simulink model "SailingYachtModel3"  (R2014a)
settings: Solver=ode3  StartTime=0.0  StopTime=40  FixedStep=0.1  RelTol=1e-3
values from neighbouring files (symbols this model uses):
  alphacoeff_xdata = alphacoeff_xdata2    [param.m]
  alphacoeff_yddata = interp1(alphacoeff_xdata,alphacoeff_yddata,alphacoeff_xdata2,'pchip')    [param.m]
  alphacoeff_yldata = interp1(alphacoeff_xdata,alphacoeff_yldata,alphacoeff_xdata2,'pchip')    [param.m]
  hull_xdata = hull_xdata2    [param.m]
  hull_ydata = arrayfun(@(x)resistancehull(x),hull_xdata2)    [param.m]
  keelcoeff_xdata = keelcoeff_xdata2    [param.m]
  keelcoeff_yddata = interp1(keelcoeff_xdata,keelcoeff_yddata,keelcoeff_xdata2,'pchip')    [param.m]
  keelcoeff_yldata = interp1(keelcoeff_xdata,keelcoeff_yldata,keelcoeff_xdata2,'pchip')    [param.m]
  ruddercoeff_xdata = ruddercoeff_xdata2    [param.m]
  ruddercoeff_yddata = arrayfun(@(x)ruddercoef_cdr(x),ruddercoeff_xdata2)    [param.m]
  ruddercoeff_yldata = interp1(ruddercoeff_xdata,ruddercoeff_yldata,ruddercoeff_xdata2,'pchip')    [param.m]
undefined symbols (not defined in the file or in its folder): par
libraries: vrlib x1
settings Model: Creator=Administrator  LastModifiedBy=paul
settings DataIOCC: SignalLoggingSaveFormat=ModelDataLogs
settings OptimizationCC: ExpressionDepthLimit=2147483647  InitFltsAndDblsToZero=on
settings DebuggingCC: SaveWithParameterizedLinksMsg=none  UnderspecifiedInitializationDetection=Classic  SignalResolutionControl=TryResolveAllWithWarning  MultiTaskDSMMsg=warning  MultiTaskCondExecSysMsg=none  FcnCallInpInsideContextMsg=UseLocalSettings  StateNameClashWarn=warning
settings RTWCC: GenCodeOnly=on  BuildConfiguration=Faster Runs  IncludeERTFirstTime=on
settings GRTTargetCC: TargetFcnLib=ansi_tfl_tmw.mat  CombineOutputUpdateFcns=off  GRTInterface=on

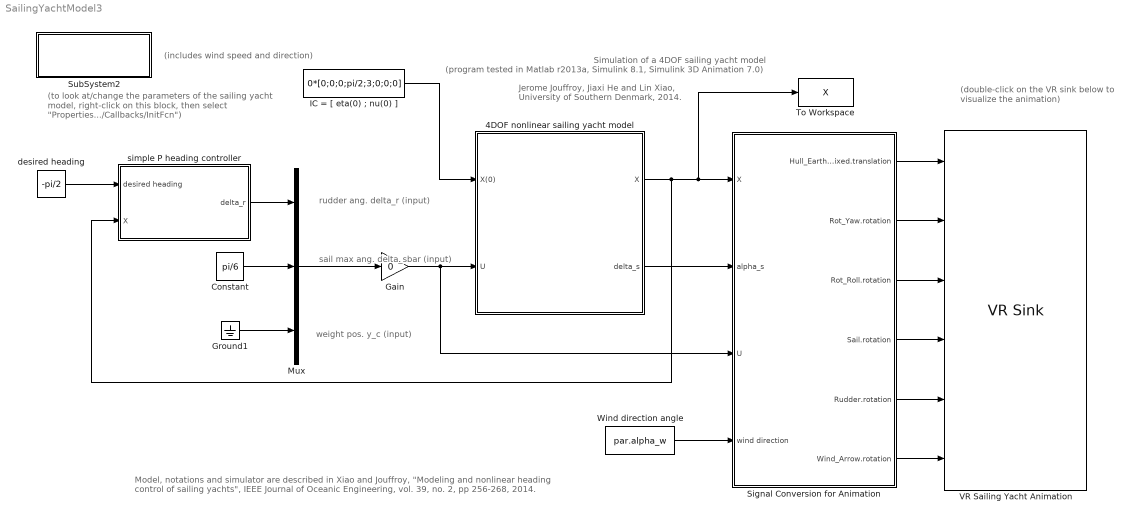
== system SailingYachtModel3 ==
  note: (includes wind speed and direction)
  note: (program tested in Matlab r2013a, Simulink 8.1, Simulink 3D Animation 7.0)
  note: (double-click on the VR sink below
      | to visualize the animation)
  note: Jerome Jouffroy, Jiaxi He and Lin Xiao,
      | University of Southern Denmark, 2014.
  note: Model, notations and simulator are described in Xiao and Jouffroy, "Modeling and nonlinear heading control of sailing yachts",
      | IEEE Journal of Oceanic Engineering, vol. 39, no. 2, pp 256-268, 2014.
  note: (to look at/change the parameters of the sailing yacht
      | model, right-click on this block, then select
      | "Properties.../Callbacks/InitFcn")
  note: weight pos. y_c (input)
  note: rudder ang. delta_r (input)
  note: sail max ang. delta_sbar (input)
  note: Simulation of a 4DOF sailing yacht model
  4DOF nonlinear sailing yacht model : Subsystem
  Constant : Constant  Value=pi/6
  Gain : Gain  Gain=0
  Ground1 : Ground
  IC = [ eta(0) ; nu(0) ] : Constant  Value=0*[0;0;0;pi/2;3;0;0;0]
  Mux : Mux  Inputs=3
  Signal Conversion for Animation : Subsystem
  SubSystem2 : Subsystem  InitFcn=|
      | global par
      | par.m = 25900;                         % (kg),mass of the vehicle
      | par.Ixx = 133690;          
      | par.Izz = 24760;      
      | par.Ixz = 2180;                        % moment of inertia
      | par.a11 = 970;   
      | par.a22 = 17430; 
      | par.a44 = 106500;
      | par.a66 = 101650;
      | par.a24 = -13160;
      | par.a26 = -6190; 
      | par.a46 = 4730;                        % (kg),added mass coef.
      | 
      | par.vt = 10;                           % the norm of wind velocity
      | par.alpha_w = pi;                      % the direction of wind (coming from the north, ie going south)
      | 
      | par.rho_a = 1.2;                       % (kg/m^3), air density
      | par.As = 170;                          % (m^2), sail area
      | par.h0 = 0.0005;                       % (m), roughness height
      | par.h1 = 11.58;                        % (m), reference height
      | par.z_s = -11.58;                      % (m), (x,y,z) is the CoE
      | par.xs = 0;
      | par.ys = 0;
      | par.zs = -11.58;                       % (m), (x,y,z) is the CoE
      | par.Xce = 0.6;                         % (m), distance along the mast to the CoE
      | par.Xm = 0.3;                          % (m), x-coordinate of the mast 
      | 
      | par.rho_w = 1025;                      % (kg/m^3), water density
      | par.Ar = 1.17;                         % (m^2), rudder area
      | par.d_r = 1.9;                         % rudder draft
      | par.zeta_r = 0.8;                      % rudder efficiency
      | par.x_r = -8.2;
      | par.z_r = -0.78;                       % (m), (x,y,z) is the CoE
      | par.xr = -8.2;
      | par.yr = 0;
      | par.zr = -0.78;                        % (m), (x,y,z) is the CoE
      | 
      | par.Ak = 8.7;                          % (m^2), keel area
      | par.d_k = 2.49;                        % keel draft
      | par.zeta_k = 0.7;                      % keel efficiency
      | par.x_k = 0;
      | par.z_k = -0.58;                       % (m), (x,y,z) is the CoE
      | par.xk = 0;
      | par.yk = 0;
      | par.zk = -0.58;                        % (m), (x,y,z) is the CoE
      | 
      | par.x_h = 0;
      | par.z_h = -1.18;                       % (m), (x,y,z) is the CoE
      | par.xh = 0;
      | par.yh = 0;
      | par.zh = -1.18;                        % (m), (x,y,z) is the CoE
      | 
      | par.w_c = 60000;                       % (N), crew weight 20000
      | par.x_c = -8;                          % (m), crew position
      | par.y_bm = 3.6;                        % (m), yacht beam
      | 
      | par.a = -5.89;
      | par.b = 8160;
      | par.c = 120000;
      | par.d = 50000;
      mask Display: disp('Parameter Initialization')
  To Workspace : ToWorkspace  VariableName=X  SaveFormat=Structure With Time  SampleTime=-1
  VR Sailing Yacht Animation : vrlib/VR Sink  InstantiateOnLoad=on  SampleTime=-1  ViewEnable=on  RemoteChange=off  RemoteView=off  FieldsWritten=Hull_EarthFixed.translation.3.1.1.double#Rot_Yaw.rotation.4.1.1.double#Rot_Roll.rotation.4.1.1.double#Sail.rotation.4.1.1.double#Rudder.rotation.4.1.1.double#Wind_Arrow.rotation.4.1.1.double  WorldFileName=SailingYachtAnimation.wrl  WorldDescription=Sailing Yacht VR animation  AutoView=on  VideoDimensions=[]  AllowVariableSize=off  FigureProperties="{'Position', 'Name', 'Viewpoint', 'CameraBound', 'CameraDirection', 'CameraPosition', 'CameraUpVector', 'ZoomFactor', 'Antialiasing', 'Headlight', 'Lighting', 'NavPanel', 'StatusBar', 'ToolBar', 'Textures', 'Transparency', 'Triad', 'Wireframe', 'NavZones', 'NavMode', 'NavSpeed', 'CaptureFileFormat', 'CaptureFileName', 'Record2DCompressMethod', 'Record2DCompressQuality', 'Record2D', 'Record2DFileName', 'Record2DFPS'; [2.0000000000000000e+00   8.0000000000000000e+01   7.9800000000000000e+02   7.1400000000000000e+02], 'Sailing Yacht VR animation', 'West', 'on', [0.0000000000000000e+00   0.0000000000000000e+00  -1.0000000000000000e+00], [0.0000000000000000e+00   0.0000000000000000e+00   0.0000000000000000e+00], [0.0000000000000000e+00   1.0000000000000000e+00   0.0000000000000000e+00], [1.0000000000000000e+00], 'on', 'on', 'on', 'halfbar', 'on', 'on', 'on', 'on', 'none', 'off', 'off', 'fly', 'normal', 'tif', '%f_anim_%n.tif', 'auto', [7.5000000000000000e+01], 'off', '%f_anim_%n.avi', 'auto'}"
  Wind direction angle : Constant  Value=par.alpha_w
  desired heading : Constant  Value=-pi/2
  simple P heading controller : Subsystem
  wires:
  Constant/1 -> Mux/2
  IC = [ eta(0) ; nu(0) ]/1 -> 4DOF nonlinear sailing yacht model/1(X(0))
  Mux/1 -> Gain/1
  4DOF nonlinear sailing yacht model/1(X) -> Signal Conversion for Animation/1(X), To Workspace/1, simple P heading controller/2(X)
  simple P heading controller/1(delta_r) -> Mux/1
  Ground1/1 -> Mux/3
  desired heading/1 -> simple P heading controller/1(desired heading)
  4DOF nonlinear sailing yacht model/2(delta_s) -> Signal Conversion for Animation/2(alpha_s)
  Wind direction angle/1 -> Signal Conversion for Animation/4(wind direction)
  Signal Conversion for Animation/1(Hull_EarthFixed.translation) -> VR Sailing Yacht Animation/1
  Signal Conversion for Animation/2(Rot_Yaw.rotation) -> VR Sailing Yacht Animation/2
  Signal Conversion for Animation/4(Sail.rotation) -> VR Sailing Yacht Animation/4
  Signal Conversion for Animation/3(Rot_Roll.rotation) -> VR Sailing Yacht Animation/3
  Signal Conversion for Animation/5(Rudder.rotation) -> VR Sailing Yacht Animation/5
  Signal Conversion for Animation/6(Wind_Arrow.rotation) -> VR Sailing Yacht Animation/6
  Gain/1 -> Signal Conversion for Animation/3(U), 4DOF nonlinear sailing yacht model/2(U)

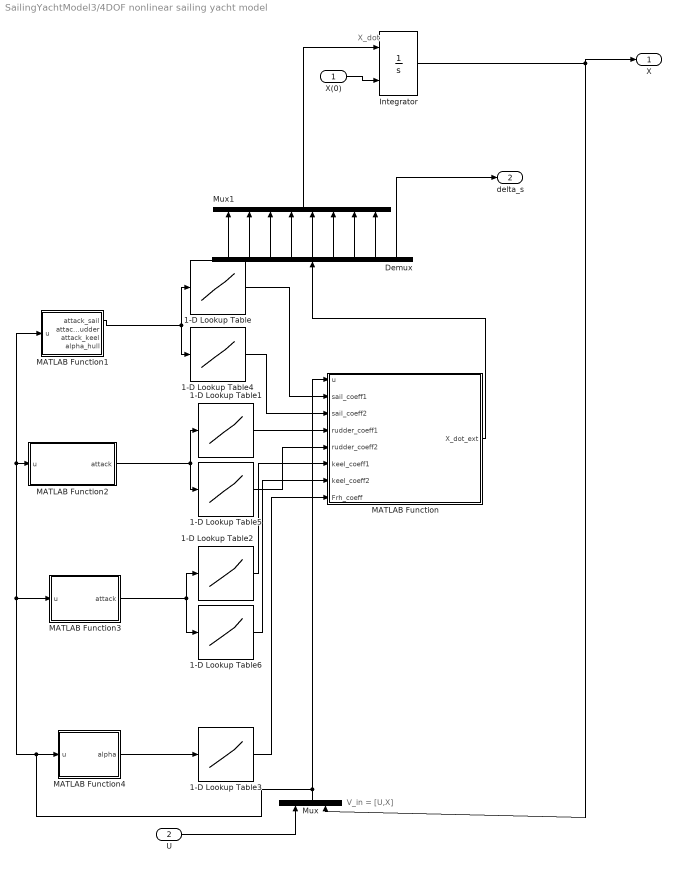
== system SailingYachtModel3/4DOF nonlinear sailing yacht model ==
  note: X_dot
  note: V_in = [U,X]
  X(0) : Inport
  U : Inport  Port=2
  1-D Lookup Table : Lookup_n-D  NumberOfTableDimensions=1  BreakpointsForDimension1=alphacoeff_xdata  Table=alphacoeff_yldata  InterpMethod=Cubic spline  RndMeth=Simplest  InputSameDT=on
  1-D Lookup Table1 : Lookup_n-D  NumberOfTableDimensions=1  BreakpointsForDimension1=ruddercoeff_xdata  Table=ruddercoeff_yldata  InterpMethod=Cubic spline  RndMeth=Simplest  InputSameDT=on
  1-D Lookup Table2 : Lookup_n-D  NumberOfTableDimensions=1  BreakpointsForDimension1=keelcoeff_xdata  Table=keelcoeff_yldata  InterpMethod=Cubic spline  DiagnosticForOutOfRangeInput=Warning  RndMeth=Simplest  InputSameDT=on
  1-D Lookup Table3 : Lookup_n-D  NumberOfTableDimensions=1  BreakpointsForDimension1=hull_xdata  Table=hull_ydata  RndMeth=Simplest  InputSameDT=on
  1-D Lookup Table4 : Lookup_n-D  NumberOfTableDimensions=1  BreakpointsForDimension1=alphacoeff_xdata  Table=alphacoeff_yddata  InterpMethod=Cubic spline  RndMeth=Simplest  InputSameDT=on
  1-D Lookup Table5 : Lookup_n-D  NumberOfTableDimensions=1  BreakpointsForDimension1=ruddercoeff_xdata  Table=ruddercoeff_yddata  InterpMethod=Cubic spline  RndMeth=Simplest  InputSameDT=on
  1-D Lookup Table6 : Lookup_n-D  NumberOfTableDimensions=1  BreakpointsForDimension1=keelcoeff_xdata  Table=keelcoeff_yddata  InterpMethod=Cubic spline  RndMeth=Simplest  InputSameDT=on
  Demux : Demux  Outputs=9
  Integrator : Integrator  InitialConditionSource=external  InitialCondition=[0;0;0;pi;1;0;0;0]
  MATLAB Function : MATLAB Function  TreatAsAtomicUnit=on
  MATLAB Function1 : MATLAB Function  TreatAsAtomicUnit=on
  MATLAB Function2 : MATLAB Function  TreatAsAtomicUnit=on
  MATLAB Function3 : MATLAB Function  TreatAsAtomicUnit=on
  MATLAB Function4 : MATLAB Function  TreatAsAtomicUnit=on
  Mux : Mux  Inputs=2
  Mux1 : Mux  Inputs=8
  X : Outport
  delta_s : Outport  Port=2
  wires:
  X(0)/1 -> Integrator/2
  Mux/1 -> MATLAB Function/1(u), MATLAB Function3/1(u), MATLAB Function2/1(u), MATLAB Function1/1(u), MATLAB Function4/1(u)
  U/1 -> Mux/1
  Integrator/1 -> X/1, Mux/2
  MATLAB Function/1(X_dot_ext) -> Demux/1
  Demux/9 -> delta_s/1
  Demux/8 -> Mux1/8
  Demux/7 -> Mux1/7
  Demux/6 -> Mux1/6
  Demux/5 -> Mux1/5
  Demux/4 -> Mux1/4
  Demux/3 -> Mux1/3
  Demux/2 -> Mux1/2
  Demux/1 -> Mux1/1
  Mux1/1 -> Integrator/1
  MATLAB Function1/1(attack_sail) -> 1-D Lookup Table/1, 1-D Lookup Table4/1
  1-D Lookup Table/1 -> MATLAB Function/2(sail_coeff1)
  MATLAB Function2/1(attack) -> 1-D Lookup Table5/1, 1-D Lookup Table1/1
  1-D Lookup Table1/1 -> MATLAB Function/4(rudder_coeff1)
  MATLAB Function3/1(attack) -> 1-D Lookup Table2/1, 1-D Lookup Table6/1
  MATLAB Function4/1(alpha) -> 1-D Lookup Table3/1
  1-D Lookup Table3/1 -> MATLAB Function/8(Frh_coeff)
  1-D Lookup Table4/1 -> MATLAB Function/3(sail_coeff2)
  1-D Lookup Table5/1 -> MATLAB Function/5(rudder_coeff2)
  1-D Lookup Table6/1 -> MATLAB Function/7(keel_coeff2)
  1-D Lookup Table2/1 -> MATLAB Function/6(keel_coeff1)

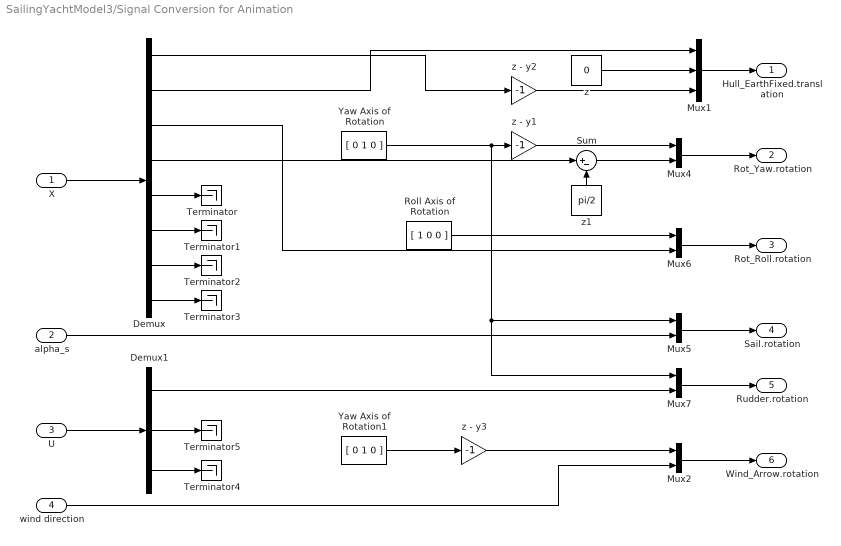
== system SailingYachtModel3/Signal Conversion for Animation ==
  X : Inport
  alpha_s : Inport  Port=2
  U : Inport  Port=3
  wind direction : Inport  Port=4
  Demux : Demux  Outputs=8
  Demux1 : Demux  Outputs=3
  Mux1 : Mux  Inputs=3
  Mux{2,4..7} (5 alike) : Mux  Inputs=2
  Roll Axis of Rotation : Constant  Value=[ 1 0 0 ]
  Sum : Sum  Inputs=|+-  SaturateOnIntegerOverflow=on
  Terminator{,1..5} (6 alike) : Terminator
  Yaw Axis of Rotation : Constant  Value=[ 0 1 0 ]
  Yaw Axis of Rotation1 : Constant  Value=[ 0 1 0 ]
  z : Constant  Value=0
  z - y1 : Gain  Gain=-1
  z - y2 : Gain  Gain=-1
  z - y3 : Gain  Gain=-1
  z1 : Constant  Value=pi/2
  Hull_EarthFixed.translation : Outport
  Rot_Yaw.rotation : Outport  Port=2
  Rot_Roll.rotation : Outport  Port=3
  Sail.rotation : Outport  Port=4
  Rudder.rotation : Outport  Port=5
  Wind_Arrow.rotation : Outport  Port=6
  wires:
  Demux/4 -> Sum/1
  Yaw Axis of Rotation/1 -> Mux5/1, Mux7/1, z - y1/1
  Sum/1 -> Mux4/2
  Roll Axis of Rotation/1 -> Mux6/1
  Demux/3 -> Mux6/2
  alpha_s/1 -> Mux5/2
  Demux/1 -> z - y2/1
  z - y2/1 -> Mux1/3
  Demux/2 -> Mux1/1
  z/1 -> Mux1/2
  z - y1/1 -> Mux4/1
  z1/1 -> Sum/2
  Mux1/1 -> Hull_EarthFixed.translation/1
  Demux/5 -> Terminator/1
  Demux/6 -> Terminator1/1
  Demux/7 -> Terminator2/1
  Demux/8 -> Terminator3/1
  X/1 -> Demux/1
  Demux1/3 -> Terminator4/1
  Demux1/2 -> Terminator5/1
  U/1 -> Demux1/1
  Demux1/1 -> Mux7/2
  Mux7/1 -> Rudder.rotation/1
  Mux5/1 -> Sail.rotation/1
  Mux4/1 -> Rot_Yaw.rotation/1
  Yaw Axis of Rotation1/1 -> z - y3/1
  z - y3/1 -> Mux2/1
  wind direction/1 -> Mux2/2
  Mux2/1 -> Wind_Arrow.rotation/1
  Mux6/1 -> Rot_Roll.rotation/1

== system SailingYachtModel3/SubSystem2 ==

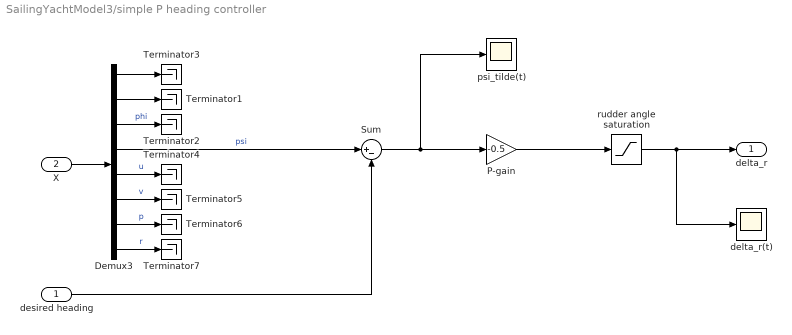
== system SailingYachtModel3/simple P heading controller ==
  desired heading : Inport
  X : Inport  Port=2
  Demux3 : Demux  Outputs=8
  P-gain : Gain  Gain=-0.5
  Sum : Sum  Inputs=|+-  SaturateOnIntegerOverflow=on
  Terminator{1..7} (7 alike) : Terminator
  delta_r(t) : Scope
      settings: YMin=-1.1  YMax=0
  psi_tilde(t) : Scope
      settings: YMin=5.55112e-17  YMax=1.6
  rudder angle saturation : Saturate  UpperLimit=pi/3  LowerLimit=-pi/3  LinearizeAsGain=off
  delta_r : Outport
  wires:
  Demux3/4 -> Sum/1  "psi"
  X/1 -> Demux3/1
  Demux3/1 -> Terminator3/1
  Demux3/2 -> Terminator1/1
  Demux3/3 -> Terminator2/1  "phi"
  Demux3/5 -> Terminator4/1  "u"
  Demux3/6 -> Terminator5/1  "v"
  Demux3/7 -> Terminator6/1  "p"
  Demux3/8 -> Terminator7/1  "r"
  Sum/1 -> psi_tilde(t)/1, P-gain/1
  P-gain/1 -> rudder angle saturation/1
  rudder angle saturation/1 -> delta_r(t)/1, delta_r/1
  desired heading/1 -> Sum/2

== matlab function SailingYachtModel3/4DOF nonlinear sailing yacht model/MATLAB Function1 ==
  data: u input; attack_sail output; attack_rudder output; attack_keel output; alpha_hull output
% interpreted Matlab function "f.m" for the Simulink file "SailingYachtModel.slx"
% This function describes the dynamics of a 4DOF sailing yacht model
% and gives the derivative of the state X and the sail angle delta_s.
% The input vector V_in contains the system state and the control input vector. 
%
% For the model description, notations, equations and parameters,
% see Xiao and Jouffroy, "Modeling and nonlinear heading control of sailing
% yachts", IEEE Journal of Oceanic Engineering, vol. 39, no. 2., pp. 256-268, 2014.
% 
% Jerome Jouffroy, Jiaxi He and Lin Xiao, 2014.
% University of Southern Denmark.



function [attack_sail,attack_rudder,attack_keel,alpha_hull]=sailcoeff_attack(u)
%#codegen

% use the system parameters
par = modeleBoat();

V_in = u;
% retrieve the system state from the field input vector "V_in"
x = V_in(5);
y = V_in(6);
phi = V_in(7);
psi = V_in(8);
u = V_in(9);
v = V_in(10);
p = V_in(11);
r = V_in(12);
nu = [ u ; v ; p ; r ];

% retrieve the input signals from the vector "V_in"
delta_r = V_in(1);
delta_sbar = V_in(2);
y_w = V_in(3);
u_s = V_in(4);


% evaluate the matrix M and C in the model
M_RB = [ par.m 0 0 0 ; 0 par.m 0 0 ; 0 0 par.Ixx -par.Ixz ; 0 0 -par.Ixz par.Izz];
C_RB = [0 -par.m*r 0 0 ; par.m*r 0 0 0 ; 0 0 0 0 ; 0 0 0 0];

M_A = [par.a11 0 0 0;0 par.a22 par.a24 par.a26;0 par.a24 par.a44 par.a46;0 par.a26 par.a46 par.a66];
C_A = [0  0 0 -par.a22*nu(2)-par.a24*nu(3)-par.a26*nu(4) ; 0 0 0 par.a11*nu(1) ; 0 0 0 0 ; par.a22*nu(2)+par.a24*nu(3)+par.a26*nu(4) -par.a11*nu(1) 0 0];

M = M_RB + M_A;

% calculate the tau vector, ie forces and moments generated from:
% the sail
v_t = [ par.vt*cos(par.alpha_w); par.vt*sin(par.alpha_w); 0 ];
v_tw = log(abs(par.z_s)*cos(phi)/par.h0)/log(par.h1/par.h0)*v_t;
R1 = [ cos(-psi) -sin(-psi) 0; sin(-psi) cos(-psi) 0; 0 0 1];
R2 = [ 1 0 0 ; 0 cos(-phi) -sin(-phi); 0 sin(-phi) cos(-phi)];
v_tb = R2*R1*v_tw; % wind expressed in the body frame
V_in = [ u ; v ; 0 ];
V_awb = v_tb - V_in - cross([p;0;r],[par.xs;par.ys;par.zs]);
V_awu = V_awb(1);
V_awv = V_awb(2);
alpha_aw = atan2(V_awv,-V_awu);

%% (sail luffing or not)
if alpha_aw-u_s>delta_sbar
    delta_s = delta_sbar;
elseif alpha_aw-u_s<-delta_sbar
    delta_s = -delta_sbar;
else
    delta_s = alpha_aw-u_s;
end
delta_s = delta_s + u_s;

alpha_as = alpha_aw - delta_s;

attack_sail = alpha_as;

% fit the input angle of attack into the interval [-pi,pi]
if attack_sail > pi
    attack_sail = mod(attack_sail+pi,2*pi) - pi;
else
    if attack_sail < -pi
        attack_sail = mod(attack_sail-pi,-2*pi) + pi;
    end
end

%% the rudder
v_aru = -u+r*par.yr;
v_arv = -v-r*par.xr + p*par.zr;
alpha_ar = atan2(v_arv,-v_aru);
alpha_a = alpha_ar-delta_r;

attack_rudder = alpha_a;

% fit the input angle of attack into the interval [-pi,pi]
if attack_rudder > pi
    attack_rudder = mod(attack_rudder+pi,2*pi) - pi;
else
    if attack_rudder < -pi
        attack_rudder = mod(attack_rudder-pi,-2*pi) + pi;
    end
end

%% the keel
v_aku = -u + r*par.yk;
v_akv = -v - r*par.xk+p*par.zk;
alpha_ak = atan2(v_akv,-v_aku);
alpha_e = alpha_ak;

attack_keel = alpha_e;

% fit the input angle of attack into the interval [-pi,pi]
if attack_keel > pi
    attack_keel = mod(attack_keel+pi,2*pi) - pi;
else
    if attack_keel < -pi
        attack_keel = mod(attack_keel-pi,-2*pi) + pi;
    end
end

%% from the hull
v_ahu = -u + r*par.yh;
v_ahv = (-v-r*par.xh + p*par.zh)/cos(phi);
v_ah = sqrt(v_aku^2+v_akv^2);
alpha_ah = atan2(v_ahv,-v_ahu);
alpha_hull = v_ah;

== matlab function SailingYachtModel3/4DOF nonlinear sailing yacht model/MATLAB Function ==
  data: u input; X_dot_ext output; sail_coeff1 input; sail_coeff2 input; rudder_coeff1 input; rudder_coeff2 input; keel_coeff1 input; keel_coeff2 input; Frh_coeff input
% interpreted Matlab function "f.m" for the Simulink file "SailingYachtModel.slx"
% This function describes the dynamics of a 4DOF sailing yacht model
% and gives the derivative of the state X and the sail angle delta_s.
% The input vector V_in contains the system state and the control input vector. 
%
% For the model description, notations, equations and parameters,
% see Xiao and Jouffroy, "Modeling and nonlinear heading control of sailing
% yachts", IEEE Journal of Oceanic Engineering, vol. 39, no. 2., pp. 256-268, 2014.
% 
% Jerome Jouffroy, Jiaxi He and Lin Xiao, 2014.
% University of Southern Denmark.



function X_dot_ext  =fcn(u,sail_coeff1,sail_coeff2,rudder_coeff1,rudder_coeff2,keel_coeff1,keel_coeff2,Frh_coeff)
%#codegen

% use the system parameters
par = modeleBoat();

V_in = u;
% retrieve the system state from the field input vector "V_in"
x = V_in(4);
y = V_in(5);
phi = V_in(6);
psi = V_in(7);
u = V_in(8);
v = V_in(9);
p = V_in(10);
r = V_in(11);
nu = [ u ; v ; p ; r ];

% retrieve the input signals from the vector "V_in"
delta_r = V_in(1);
delta_sbar = V_in(2);
y_w = V_in(3);

% evaluate the matrix M and C in the model
M_RB = [ par.m 0 0 0 ; 0 par.m 0 0 ; 0 0 par.Ixx -par.Ixz ; 0 0 -par.Ixz par.Izz];
C_RB = [0 -par.m*r 0 0 ; par.m*r 0 0 0 ; 0 0 0 0 ; 0 0 0 0];

M_A = [par.a11 0 0 0;0 par.a22 par.a24 par.a26;0 par.a24 par.a44 par.a46;0 par.a26 par.a46 par.a66];
C_A = [0  0 0 -par.a22*nu(2)-par.a24*nu(3)-par.a26*nu(4) ; 0 0 0 par.a11*nu(1) ; 0 0 0 0 ; par.a22*nu(2)+par.a24*nu(3)+par.a26*nu(4) -par.a11*nu(1) 0 0];

M = M_RB + M_A;

% calculate the tau vector, ie forces and moments generated from:
% the sail
v_t = [ par.vt*cos(par.alpha_w); par.vt*sin(par.alpha_w); 0 ];
v_tw = log(abs(par.z_s)*cos(phi)/par.h0)/log(par.h1/par.h0)*v_t;
R1 = [ cos(-psi) -sin(-psi) 0; sin(-psi) cos(-psi) 0; 0 0 1];
R2 = [ 1 0 0 ; 0 cos(-phi) -sin(-phi); 0 sin(-phi) cos(-phi)];
v_tb = R2*R1*v_tw; % wind expressed in the body frame
V_in = [ u ; v ; 0 ];
V_awb = v_tb - V_in - cross([p;0;r],[par.xs;par.ys;par.zs]);
V_awu = V_awb(1);
V_awv = V_awb(2);
alpha_aw = atan2(V_awv,-V_awu);

% (sail luffing or not)
if alpha_aw>delta_sbar
    delta_s = delta_sbar;
elseif alpha_aw<-delta_sbar
    delta_s = -delta_sbar;
else
    delta_s = alpha_aw;
end

alpha_as = alpha_aw - delta_s;

Cls = sail_coeff1;
Cds = sail_coeff2;

Ls = 0.5*par.rho_a*par.As*(V_awu^2+V_awv^2)*Cls;
Ds = 0.5*par.rho_a*par.As*(V_awu^2+V_awv^2)*Cds;

tau_sail = [Ls*sin(alpha_aw)-Ds*cos(alpha_aw); Ls*cos(alpha_aw)+Ds*sin(alpha_aw);-(Ls*cos(alpha_aw)+Ds*sin(alpha_aw))*par.zs; -(Ls*sin(alpha_aw)-Ds*cos(alpha_aw))*par.Xce*sin(delta_s)+(Ls*cos(alpha_aw)+Ds*sin(alpha_aw))*(par.Xm-par.Xce*cos(delta_s))];
Mzs = tau_sail(4);

% the rudder
v_aru = -u+r*par.yr;
v_arv = -v-r*par.xr + p*par.zr;
alpha_ar = atan2(v_arv,-v_aru);
alpha_a = alpha_ar-delta_r;

%[Clr,Cdr] = ruddercoef(alpha_a);
Clr = rudder_coeff1;
Cdr = rudder_coeff2;

Cdr = Cdr+Clr^2*par.Ar/(pi*2*par.zeta_r*par.d_r^2);

Lr = 0.5*par.rho_w*par.Ar*(v_aru^2+v_arv^2)*Clr;
Dr = 0.5*par.rho_w*par.Ar*(v_aru^2+v_arv^2)*Cdr;

tau_rudder = [Lr*sin(alpha_ar)-Dr*cos(alpha_ar); Lr*cos(alpha_ar)+Dr*sin(alpha_ar); -(Lr*cos(alpha_ar)+Dr*sin(alpha_ar))*par.zr; (Lr*cos(alpha_ar)+Dr*sin(alpha_ar))*par.xr];
Mzr = tau_rudder(4);

% the tau vector is finally given by:
tau = tau_sail + tau_rudder;

% calculate the damping forces and moments:
% from the keel
v_aku = -u + r*par.yk;
v_akv = -v - r*par.xk+p*par.zk;
alpha_ak = atan2(v_akv,-v_aku);
alpha_e = alpha_ak;

Clk = keel_coeff1;
Cdk = keel_coeff2;

Cdk = Cdk + Clk^2*par.Ak/(pi*2*par.zeta_k*par.d_k^2);

Lk = 0.5*par.rho_w*par.Ak*(v_aku^2+v_akv^2)*Clk;
Dk = 0.5*par.rho_w*par.Ak*(v_aku^2+v_akv^2)*Cdk;

D_keel = [ -Lk*sin(alpha_ak)+Dk*cos(alpha_ak); -Lk*cos(alpha_ak)-Dk*sin(alpha_ak); -(-Lk*cos(alpha_ak)-Dk*sin(alpha_ak))*par.zk; -(Lk*cos(alpha_ak)+Dk*sin(alpha_ak))*par.xk];

% from the hull
v_ahu = -u + r*par.yh;
v_ahv = (-v-r*par.xh + p*par.zh)/cos(phi);
v_ah = sqrt(v_aku^2+v_akv^2);
alpha_ah = atan2(v_ahv,-v_ahu);

Frh = Frh_coeff;

D_hull = [Frh*cos(alpha_ah);-Frh*sin(alpha_ah)*cos(phi); Frh*sin(alpha_ah)*cos(phi)*par.zh; -Frh*sin(alpha_ah)*cos(phi)*par.xh];

% from heel and yaw
% (compute first eta_dot and thereby phi_dot and psi_dot)
J = [cos(psi) -sin(psi)*cos(phi) 0 0; sin(psi) cos(psi)*cos(phi) 0 0; 0 0 1 0; 0 0 0 cos(phi)];
eta_dot = J*nu;
phi_dot = eta_dot(3);
psi_dot = eta_dot(4);

D_heelandyaw = [0;0;par.c*phi_dot*abs(phi_dot);par.d*psi_dot*abs(psi_dot)*cos(phi)]; 

% compute total damping vector D
D = D_keel + D_hull + D_heelandyaw;

% righting moment plus internal moving mass system (ie transversal weight)
phi_deg = phi*180/pi;
M_xw = -y_w*par.w_c*par.y_bm*cos(phi);
M_zw = -y_w*par.w_c*par.x_c*sin(abs(phi));
G = [ 0 ; 0 ; par.a*phi_deg^2+par.b*phi_deg + M_xw ; M_zw];

% computation of nu_dot
nu_dot = -M\(C_RB*nu+C_A*nu)-M\D-M\G+M\tau; 
 

% output the derivative of the state extended with the sail angle
X_dot_ext = [ eta_dot   ; 
              nu_dot   ;
              delta_s];

== matlab function SailingYachtModel3/4DOF nonlinear sailing yacht model/MATLAB Function2 ==
  data: u input; attack output
% interpreted Matlab function "f.m" for the Simulink file "SailingYachtModel.slx"
% This function describes the dynamics of a 4DOF sailing yacht model
% and gives the derivative of the state X and the sail angle delta_s.
% The input vector V_in contains the system state and the control input vector. 
%
% For the model description, notations, equations and parameters,
% see Xiao and Jouffroy, "Modeling and nonlinear heading control of sailing
% yachts", IEEE Journal of Oceanic Engineering, vol. 39, no. 2., pp. 256-268, 2014.
% 
% Jerome Jouffroy, Jiaxi He and Lin Xiao, 2014.
% University of Southern Denmark.



function attack=ruddercoeff_attack(u)
%#codegen

% use the system parameters
par = modeleBoat();


V_in = u;
% retrieve the system state from the field input vector "V_in"
x = V_in(4);
y = V_in(5);
phi = V_in(6);
psi = V_in(7);
u = V_in(8);
v = V_in(9);
p = V_in(10);
r = V_in(11);
nu = [ u ; v ; p ; r ];

% retrieve the input signals from the vector "V_in"
delta_r = V_in(1);
delta_sbar = V_in(2);
y_w = V_in(3);

% evaluate the matrix M and C in the model
M_RB = [ par.m 0 0 0 ; 0 par.m 0 0 ; 0 0 par.Ixx -par.Ixz ; 0 0 -par.Ixz par.Izz];
C_RB = [0 -par.m*r 0 0 ; par.m*r 0 0 0 ; 0 0 0 0 ; 0 0 0 0];

M_A = [par.a11 0 0 0;0 par.a22 par.a24 par.a26;0 par.a24 par.a44 par.a46;0 par.a26 par.a46 par.a66];
C_A = [0  0 0 -par.a22*nu(2)-par.a24*nu(3)-par.a26*nu(4) ; 0 0 0 par.a11*nu(1) ; 0 0 0 0 ; par.a22*nu(2)+par.a24*nu(3)+par.a26*nu(4) -par.a11*nu(1) 0 0];

M = M_RB + M_A;

% calculate the tau vector, ie forces and moments generated from:
% the sail
v_t = [ par.vt*cos(par.alpha_w); par.vt*sin(par.alpha_w); 0 ];
v_tw = log(abs(par.z_s)*cos(phi)/par.h0)/log(par.h1/par.h0)*v_t;
R1 = [ cos(-psi) -sin(-psi) 0; sin(-psi) cos(-psi) 0; 0 0 1];
R2 = [ 1 0 0 ; 0 cos(-phi) -sin(-phi); 0 sin(-phi) cos(-phi)];
v_tb = R2*R1*v_tw; % wind expressed in the body frame
V_in = [ u ; v ; 0 ];
V_awb = v_tb - V_in - cross([p;0;r],[par.xs;par.ys;par.zs]);
V_awu = V_awb(1);
V_awv = V_awb(2);
alpha_aw = atan2(V_awv,-V_awu);

% (sail luffing or not)
if alpha_aw>delta_sbar
    delta_s = delta_sbar;
elseif alpha_aw<-delta_sbar
    delta_s = -delta_sbar;
else
    delta_s = alpha_aw;
end

alpha_as = alpha_aw - delta_s;


% the rudder
v_aru = -u+r*par.yr;
v_arv = -v-r*par.xr + p*par.zr;
alpha_ar = atan2(v_arv,-v_aru);
alpha_a = alpha_ar-delta_r;

attack = alpha_a;

% fit the input angle of attack into the interval [-pi,pi]
if attack > pi
    attack = mod(attack+pi,2*pi) - pi;
else
    if attack < -pi
        attack = mod(attack-pi,-2*pi) + pi;
    end
end

% interpolation
%attack = attack/pi*180;




%------------------------------------------------------------------------------------------------------------------------------
function [Clr,Cdr] = ruddercoef(attack)
% generate a lookup table for the lift/drag coefficients for the sail
% and compute Cls/Cds from the lookup table using interpolation.

% lookup table
xdata = linspace(-pi,pi,73); % every 5 degrees
xdata = xdata/pi*180;

% lift curve
yl = fliplr([0 0.42 0.73 ...
    0.95 1.1 1.165 1.18 1.155 1.12 1.065 1 0.92 0.83 0.72 0.62 0.48 0.33 0.16])*(-1);
yldata = [fliplr([0 0.42 0.73 ...
    0.95 1.1 1.165 1.18 1.155 1.12 1.065 1 0.92 0.83 0.72 0.62 0.48 0.33 0.16 0 yl])*(-1) ...
    [0.42 0.73 ...
    0.95 1.1 1.165 1.18 1.155 1.12 1.065 1 0.92 0.83 0.72 0.62 0.48 0.33 0.16 0 yl]];

% drag curve
yd = fliplr([0 0.03 0.06 ...
    0.1 0.17 0.3 0.48 0.74 0.98 1.18 1.34 1.5 1.65 1.76 1.89 1.97 2.01 2.05]);
yddata = [fliplr([0 0.03 0.06 ...
    0.1 0.17 0.3 0.48 0.74 0.98 1.18 1.34 1.5 1.65 1.76 1.89 1.97 2.01 2.05 2.08 yd])...
    [0.03 0.06 ...
    0.1 0.17 0.3 0.48 0.74 0.98 1.18 1.34 1.5 1.65 1.76 1.89 1.97 2.01 2.05 2.08 yd]];

% fit the input angle of attack into the interval [-pi,pi]
if attack > pi
    attack = mod(attack+pi,2*pi) - pi;
else
    if attack < -pi
        attack = mod(attack-pi,-2*pi) + pi;
    end
end

% interpolation
attack = attack/pi*180;
Clr = interp1(xdata,yldata,attack,'pchip');
Cdr = interp1(xdata,yddata,attack,'pchip');


%------------------------------------------------------------------------------------------------------------------------------
function [Clk,Cdk] = keelcoef(attack)
% generate a lookup table for the lift/drag coefficients for the sail
% and compute Cls/Cds from the lookup table using interpolation.

% lookup table
xdata = linspace(-pi,pi,73); % every 5 degrees
xdata = xdata/pi*180;

% lift curve
yl = fliplr([0 0.425 0.74 ...
    0.94 1.1 1.17 1.19 1.16 1.12 1.07 0.99 0.92 0.84 0.74 0.63 0.49 0.345 0.185])*(-1);
yldata = [fliplr([0 0.425 0.74 ...
    0.94 1.1 1.17 1.19 1.16 1.12 1.07 0.99 0.92 0.84 0.74 0.63 0.49 0.345 0.185 0 yl])*(-1) ...
    [0.425 0.74 ...
    0.94 1.1 1.17 1.19 1.16 1.12 1.07 0.99 0.92 0.84 0.74 0.63 0.49 0.345 0.185 0 yl]];

% drag curve
yd = fliplr([0 0.04 0.07 ...
    0.1 0.17 0.3 0.49 0.76 0.98 1.19 1.34 1.5 1.65 1.77 1.88 1.96 2.01 2.05]);
yddata = [fliplr([0 0.04 0.07 ...
    0.1 0.17 0.3 0.49 0.76 0.98 1.19 1.34 1.5 1.65 1.77 1.88 1.96 2.01 2.05 2.09 yd])...
    [0.04 0.07 ...
    0.1 0.17 0.3 0.49 0.76 0.98 1.19 1.34 1.5 1.65 1.77 1.88 1.96 2.01 2.05 2.09 yd]];

% fit the input angle of attack into the interval [-pi,pi]
if attack > pi
    attack = mod(attack+pi,2*pi) - pi;
else
    if attack < -pi
        attack = mod(attack-pi,-2*pi) + pi;
    end
end

% interpolation
attack = attack/pi*180;
Clk = interp1(xdata,yldata,attack,'pchip');
Cdk = interp1(xdata,yddata,attack,'pchip');


%------------------------------------------------------------------------------------------------------------------------------
function F = resistancehull(alpha_a)

xdata = linspace(0,6,13); % every 0.5m/s
ydata = [0 0.15 0.35 0.5 0.675 0.825 1.175 1.4 2 4.85 9.85 18.46 27.5]*1000;

% interpolation
if alpha_a <= 6
    F = interp1(xdata,ydata,alpha_a,'pchip');
else
    F = interp1(xdata,ydata,alpha_a,'pchip','extrap');
end

== matlab function SailingYachtModel3/4DOF nonlinear sailing yacht model/MATLAB Function3 ==
  data: u input; attack output
% interpreted Matlab function "f.m" for the Simulink file "SailingYachtModel.slx"
% This function describes the dynamics of a 4DOF sailing yacht model
% and gives the derivative of the state X and the sail angle delta_s.
% The input vector V_in contains the system state and the control input vector. 
%
% For the model description, notations, equations and parameters,
% see Xiao and Jouffroy, "Modeling and nonlinear heading control of sailing
% yachts", IEEE Journal of Oceanic Engineering, vol. 39, no. 2., pp. 256-268, 2014.
% 
% Jerome Jouffroy, Jiaxi He and Lin Xiao, 2014.
% University of Southern Denmark.



function attack=keelcoeff_attack(u)
%#codegen

% use the system parameters
par = modeleBoat();


V_in = u;
% retrieve the system state from the field input vector "V_in"
x = V_in(4);
y = V_in(5);
phi = V_in(6);
psi = V_in(7);
u = V_in(8);
v = V_in(9);
p = V_in(10);
r = V_in(11);
nu = [ u ; v ; p ; r ];

% retrieve the input signals from the vector "V_in"
delta_r = V_in(1);
delta_sbar = V_in(2);
y_w = V_in(3);

% evaluate the matrix M and C in the model
M_RB = [ par.m 0 0 0 ; 0 par.m 0 0 ; 0 0 par.Ixx -par.Ixz ; 0 0 -par.Ixz par.Izz];
C_RB = [0 -par.m*r 0 0 ; par.m*r 0 0 0 ; 0 0 0 0 ; 0 0 0 0];

M_A = [par.a11 0 0 0;0 par.a22 par.a24 par.a26;0 par.a24 par.a44 par.a46;0 par.a26 par.a46 par.a66];
C_A = [0  0 0 -par.a22*nu(2)-par.a24*nu(3)-par.a26*nu(4) ; 0 0 0 par.a11*nu(1) ; 0 0 0 0 ; par.a22*nu(2)+par.a24*nu(3)+par.a26*nu(4) -par.a11*nu(1) 0 0];

M = M_RB + M_A;

% calculate the tau vector, ie forces and moments generated from:
% the sail
v_t = [ par.vt*cos(par.alpha_w); par.vt*sin(par.alpha_w); 0 ];
v_tw = log(abs(par.z_s)*cos(phi)/par.h0)/log(par.h1/par.h0)*v_t;
R1 = [ cos(-psi) -sin(-psi) 0; sin(-psi) cos(-psi) 0; 0 0 1];
R2 = [ 1 0 0 ; 0 cos(-phi) -sin(-phi); 0 sin(-phi) cos(-phi)];
v_tb = R2*R1*v_tw; % wind expressed in the body frame
V_in = [ u ; v ; 0 ];
V_awb = v_tb - V_in - cross([p;0;r],[par.xs;par.ys;par.zs]);
V_awu = V_awb(1);
V_awv = V_awb(2);
alpha_aw = atan2(V_awv,-V_awu);


% calculate the damping forces and moments:
% from the keel
v_aku = -u + r*par.yk;
v_akv = -v - r*par.xk+p*par.zk;
alpha_ak = atan2(v_akv,-v_aku);
alpha_e = alpha_ak;

attack = alpha_e;

% fit the input angle of attack into the interval [-pi,pi]
if attack > pi
    attack = mod(attack+pi,2*pi) - pi;
else
    if attack < -pi
        attack = mod(attack-pi,-2*pi) + pi;
    end
end

% interpolation
%attack = attack/pi*180;

== matlab function SailingYachtModel3/4DOF nonlinear sailing yacht model/MATLAB Function4 ==
  data: u input; alpha output
% interpreted Matlab function "f.m" for the Simulink file "SailingYachtModel.slx"
% This function describes the dynamics of a 4DOF sailing yacht model
% and gives the derivative of the state X and the sail angle delta_s.
% The input vector V_in contains the system state and the control input vector. 
%
% For the model description, notations, equations and parameters,
% see Xiao and Jouffroy, "Modeling and nonlinear heading control of sailing
% yachts", IEEE Journal of Oceanic Engineering, vol. 39, no. 2., pp. 256-268, 2014.
% 
% Jerome Jouffroy, Jiaxi He and Lin Xiao, 2014.
% University of Southern Denmark.



function alpha=fcn(u)
%#codegen

% use the system parameters
par = modeleBoat();


V_in = u;
% retrieve the system state from the field input vector "V_in"
x = V_in(4);
y = V_in(5);
phi = V_in(6);
psi = V_in(7);
u = V_in(8);
v = V_in(9);
p = V_in(10);
r = V_in(11);
nu = [ u ; v ; p ; r ];

% retrieve the input signals from the vector "V_in"
delta_r = V_in(1);
delta_sbar = V_in(2);
y_w = V_in(3);

% evaluate the matrix M and C in the model
M_RB = [ par.m 0 0 0 ; 0 par.m 0 0 ; 0 0 par.Ixx -par.Ixz ; 0 0 -par.Ixz par.Izz];
C_RB = [0 -par.m*r 0 0 ; par.m*r 0 0 0 ; 0 0 0 0 ; 0 0 0 0];

M_A = [par.a11 0 0 0;0 par.a22 par.a24 par.a26;0 par.a24 par.a44 par.a46;0 par.a26 par.a46 par.a66];
C_A = [0  0 0 -par.a22*nu(2)-par.a24*nu(3)-par.a26*nu(4) ; 0 0 0 par.a11*nu(1) ; 0 0 0 0 ; par.a22*nu(2)+par.a24*nu(3)+par.a26*nu(4) -par.a11*nu(1) 0 0];

M = M_RB + M_A;

% calculate the tau vector, ie forces and moments generated from:
% the sail
v_t = [ par.vt*cos(par.alpha_w); par.vt*sin(par.alpha_w); 0 ];
v_tw = log(abs(par.z_s)*cos(phi)/par.h0)/log(par.h1/par.h0)*v_t;
R1 = [ cos(-psi) -sin(-psi) 0; sin(-psi) cos(-psi) 0; 0 0 1];
R2 = [ 1 0 0 ; 0 cos(-phi) -sin(-phi); 0 sin(-phi) cos(-phi)];
v_tb = R2*R1*v_tw; % wind expressed in the body frame
V_in = [ u ; v ; 0 ];
V_awb = v_tb - V_in - cross([p;0;r],[par.xs;par.ys;par.zs]);
V_awu = V_awb(1);
V_awv = V_awb(2);
alpha_aw = atan2(V_awv,-V_awu);

% calculate the damping forces and moments:
% from the keel
v_aku = -u + r*par.yk;
v_akv = -v - r*par.xk+p*par.zk;
alpha_ak = atan2(v_akv,-v_aku);
alpha_e = alpha_ak;

% from the hull
v_ahu = -u + r*par.yh;
v_ahv = (-v-r*par.xh + p*par.zh)/cos(phi);
v_ah = sqrt(v_aku^2+v_akv^2);
alpha_ah = atan2(v_ahv,-v_ahu);
alpha = v_ah;
